simulink model "vi_du_1_r2015a"  (R2015a)
settings: Solver=ode4  SolverMode=SingleTasking  StartTime=0.0  StopTime=80  FixedStep=0.001  RelTol=1e-3
settings Model: CovMetricSettings=dwe  CovHtmlReporting=off  covSaveCumulativeToWorkspaceVar=off  CovSaveSingleToWorkspaceVar=off  CovExternalEMLEnable=on  Creator=ryell  LastModifiedBy=ryell
settings DataIOCC: LimitDataPoints=off  SaveFormat=Dataset
settings DebuggingCC: SFUnexpectedBacktrackingDiag=error  SFNoUnconditionalDefaultTransitionDiag=error
settings HardwareCC: ProdBitPerPointer=64  ProdLargestAtomicFloat=Float  ProdIntDivRoundTo=Zero  ProdEndianess=LittleEndian  ProdHWDeviceType=Specified
settings ModelReferenceCC: PropagateSignalLabelsOutOfModel=on
settings GRTTargetCC: TargetLangStandard=C99 (ISO)  GeneratePreprocessorConditionals=Use local settings

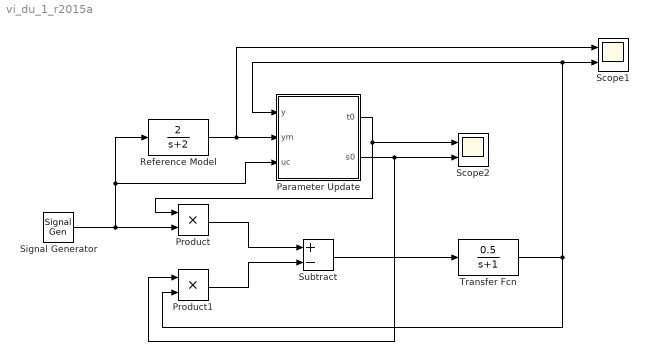
== system vi_du_1_r2015a ==
  Parameter Update : Subsystem  mask{gamma=10, t0_init=0, s0_init=0}
  Product : Product
  Product1 : Product
  Reference Model : TransferFcn  Numerator=[2]  Denominator=[1 2]
  Scope1 : Scope  NumInputPorts=2
      settings: TimeRange=auto  ShowLegends=on  MaxDataPoints=5000  SaveToWorkspace=off  SaveName=ScopeData  YMin=-2.16357~-5  YMax=2.32673~5  SampleTime=-1
  Scope2 : Scope  NumInputPorts=2
      settings: TimeRange=auto  ShowLegends=on  MaxDataPoints=5000  SaveToWorkspace=off  YMin=-0.77657~-5  YMax=5.25928~5  SampleTime=-1
  Signal Generator : SignalGenerator  WaveForm=square  Frequency=0.1
  Subtract : Sum  Inputs=+-
  Transfer Fcn : TransferFcn  Numerator=[0.5]  Denominator=[1 1]
  wires:
  Product/1 -> Subtract/1
  Product1/1 -> Subtract/2
  Subtract/1 -> Transfer Fcn/1
  Transfer Fcn/1 -> Product1/2, Scope1/2, Parameter Update/1(y)
  Parameter Update/2(s0) -> Scope2/2, Product1/1
  Signal Generator/1 -> Reference Model/1, Parameter Update/3(uc), Product/2
  Parameter Update/1(t0) -> Scope2/1, Product/1
  Reference Model/1 -> Scope1/1, Parameter Update/2(ym)

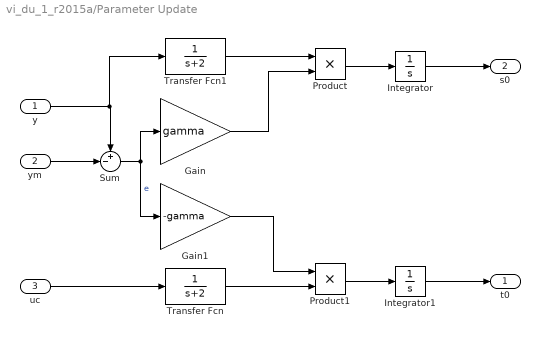
== system vi_du_1_r2015a/Parameter Update ==
  y : Inport
  ym : Inport  Port=2
  uc : Inport  Port=3
  Gain : Gain  Gain=gamma
  Gain1 : Gain  Gain=-gamma
  Integrator : Integrator  InitialCondition=t0_init
  Integrator1 : Integrator  InitialCondition=s0_init
  Product : Product
  Product1 : Product
  Sum : Sum  Inputs=+-|
  Transfer Fcn : TransferFcn  Denominator=[1 2]
  Transfer Fcn1 : TransferFcn  Denominator=[1 2]
  t0 : Outport
  s0 : Outport  Port=2
  wires:
  y/1 -> Transfer Fcn1/1, Sum/1
  ym/1 -> Sum/2
  Sum/1 -> Gain1/1, Gain/1  "e"
  uc/1 -> Transfer Fcn/1
  Transfer Fcn1/1 -> Product/1
  Transfer Fcn/1 -> Product1/2
  Gain/1 -> Product/2
  Gain1/1 -> Product1/1
  Product/1 -> Integrator/1
  Product1/1 -> Integrator1/1
  Integrator/1 -> s0/1
  Integrator1/1 -> t0/1
